simulink model "Transmission_system"  (R2015a)
settings: Solver=ode45  StartTime=0.0  StopTime=10.0  RelTol=1e-3
undefined symbols (not defined in the file): D1, Delta
libraries: powerlib x39
settings Model: Creator=Rangga Putra  LastModifiedBy=Rangga Putra

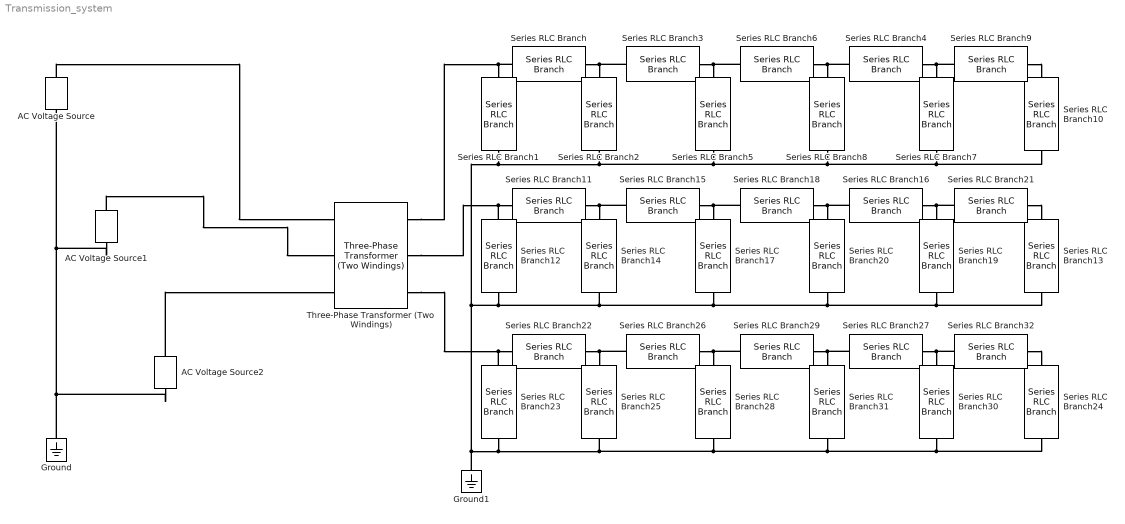
== system Transmission_system ==
  AC Voltage Source : powerlib/Electrical Sources/AC Voltage Source  Amplitude=100  Phase=0  Frequency=60  SampleTime=0  Measurements=None
  AC Voltage Source1 : powerlib/Electrical Sources/AC Voltage Source  Amplitude=100  Phase=0  Frequency=60  SampleTime=0  Measurements=None
  AC Voltage Source2 : powerlib/Electrical Sources/AC Voltage Source  Amplitude=100  Phase=0  Frequency=60  SampleTime=0  Measurements=None
  Ground : powerlib/Elements/Ground  LConnTagsString=a
  Ground1 : powerlib/Elements/Ground  LConnTagsString=a
  Series RLC Branch{,3..4,6,9,11,15..16,18,21..22,26..27,29,32} (15 alike) : powerlib/Elements/Series RLC Branch  LConnTagsString=__new0  RConnTagsString=__new0  BranchType=RL  Resistance=0.52  Inductance=2.5e-3  SetiL0=off  InitialCurrent=0  Capacitance=1e-6  Setx0=off  InitialVoltage=0  Measurements=None
  Series RLC Branch{1,10,12..13,23..24} (6 alike) : powerlib/Elements/Series RLC Branch  LConnTagsString=__new0  RConnTagsString=__new0  BranchType=C  Resistance=1  Inductance=1e-3  SetiL0=off  InitialCurrent=0  Capacitance=2.5e-6  Setx0=off  InitialVoltage=0  Measurements=None
  Series RLC Branch{2,5,7..8,14,17,19..20,25,28,30..31} (12 alike) : powerlib/Elements/Series RLC Branch  LConnTagsString=__new0  RConnTagsString=__new0  BranchType=C  Resistance=1  Inductance=1e-3  SetiL0=off  InitialCurrent=0  Capacitance=5e-6  Setx0=off  InitialVoltage=0  Measurements=None
  Three-Phase Transformer (Two Windings) : powerlib/Elements/Three-Phase Transformer (Two Windings)  Winding1Connection=Delta (D1)  Winding2Connection=Yg  CoreType=Three single-phase transformers  SetSaturation=off  Hysteresis=off  DataFile='hysteresis'  SetInitialFlux=off  Measurements=None  UNITS=pu  NominalPower=[ 250e6 , 60 ]  Winding1=[ 735e3 , 0.002 , 0.08 ]  Winding2=[ 315e3 , 0.002 , 0.08 ]  Rm=500  Lm=500  L0=0.5  Saturation=[ 0,0 ; 0.0024,1.2 ; 1.0,1.52 ]  InitialFluxes=[ 0.8 , -0.8 , 0.7 ]  MoreParameters=off  BreakLoop=off  DataType=off  TransfoNumber=1
  connections:
  Series RLC Branch/RConn1 -- Series RLC Branch3/LConn1 -- Series RLC Branch2/LConn1
  Series RLC Branch3/RConn1 -- Series RLC Branch6/LConn1 -- Series RLC Branch5/LConn1
  Series RLC Branch6/RConn1 -- Series RLC Branch4/LConn1 -- Series RLC Branch8/LConn1
  Series RLC Branch4/RConn1 -- Series RLC Branch9/LConn1 -- Series RLC Branch7/LConn1
  Series RLC Branch11/RConn1 -- Series RLC Branch15/LConn1 -- Series RLC Branch14/LConn1
  Series RLC Branch15/RConn1 -- Series RLC Branch18/LConn1 -- Series RLC Branch17/LConn1
  Series RLC Branch18/RConn1 -- Series RLC Branch16/LConn1 -- Series RLC Branch20/LConn1
  Series RLC Branch16/RConn1 -- Series RLC Branch21/LConn1 -- Series RLC Branch19/LConn1
  Series RLC Branch12/LConn1 -- Three-Phase Transformer (Two Windings)/RConn2 -- Series RLC Branch11/LConn1
  Series RLC Branch22/RConn1 -- Series RLC Branch26/LConn1 -- Series RLC Branch25/LConn1
  Series RLC Branch26/RConn1 -- Series RLC Branch29/LConn1 -- Series RLC Branch28/LConn1
  Series RLC Branch29/RConn1 -- Series RLC Branch27/LConn1 -- Series RLC Branch31/LConn1
  Series RLC Branch27/RConn1 -- Series RLC Branch32/LConn1 -- Series RLC Branch30/LConn1
  Series RLC Branch14/RConn1 -- Series RLC Branch12/RConn1 -- Series RLC Branch10/RConn1 -- Series RLC Branch7/RConn1 -- Series RLC Branch8/RConn1 -- Series RLC Branch5/RConn1 -- Series RLC Branch2/RConn1 -- Series RLC Branch1/RConn1 -- Ground1/LConn1 -- Series RLC Branch23/RConn1 -- Series RLC Branch24/RConn1 -- Series RLC Branch30/RConn1 -- Series RLC Branch31/RConn1 -- Series RLC Branch28/RConn1 -- Series RLC Branch25/RConn1 -- Series RLC Branch17/RConn1 -- Series RLC Branch20/RConn1 -- Series RLC Branch13/RConn1 -- Series RLC Branch19/RConn1
  Series RLC Branch23/LConn1 -- Three-Phase Transformer (Two Windings)/RConn3 -- Series RLC Branch22/LConn1
  AC Voltage Source/LConn1 -- AC Voltage Source2/LConn1 -- Ground/LConn1 -- AC Voltage Source1/LConn1
  Three-Phase Transformer (Two Windings)/RConn1 -- Series RLC Branch/LConn1 -- Series RLC Branch1/LConn1
  Series RLC Branch32/RConn1 -- Series RLC Branch24/LConn1
  Series RLC Branch9/RConn1 -- Series RLC Branch10/LConn1
  AC Voltage Source1/RConn1 -- Three-Phase Transformer (Two Windings)/LConn2
  AC Voltage Source2/RConn1 -- Three-Phase Transformer (Two Windings)/LConn3
  Series RLC Branch21/RConn1 -- Series RLC Branch13/LConn1
  AC Voltage Source/RConn1 -- Three-Phase Transformer (Two Windings)/LConn1
